simulink subsystem "ElectricalThermalSystem"  (R2025a)
settings: Solver=VariableStepAuto  StartTime=0.0  StopTime=10.0  RelTol=1e-3
undefined symbols (not defined in the file): EnvAirTemp, PlantThrEstCmpPwr, PlntThrAirBpt, PlntThrAirCond, PlntThrAirCp, PlntThrAirCpBpt, PlntThrAirPrand, PlntThrAirRho, PlntThrAirVisc, PlntThrBattDCFlwRatio, PlntThrBattJacLen, PlntThrChArea, PlntThrChDia, PlntThrCoolCond, PlntThrCoolCp, PlntThrCoolCpBpt, PlntThrCoolPrand, PlntThrCoolRho, PlntThrCoolVisc, PlntThrDCJacLen, PlntThrEMJacLen, PlntThrEstCOPLut, PlntThrEstDTLut, PlntThrHeaterMaxPwr, PlntThrPmpDisp, PlntThrPmpHeadP, PlntThrPmpMaxSpd, PlntThrPmpMechEff, PlntThrPmpVolEff, PlntThrRadAirArea, PlntThrRadAirDh, PlntThrRadFanAreaFlw, PlntThrRadFlwCoef, PlntThrRadGapHeight, PlntThrRadLength, PlntThrRadNTubes, PlntThrRadTubeDh, PlntThrRadTubeHeight, PlntThrRadWidth
libraries: autolibutils x62
(part 3 of 4)

== system ElectricalThermalSystem/Heater Battery DCDC Converter/DC-DC Converter/Heat-flow Rate ==
  HTC : Inport
  PwrETemp : Inport  Port=2
  JacArea : Inport  Port=3
  CoolBlkTemp : Inport  Port=4
  Product1 : Product  Inputs=3
  Subtract : Sum  Inputs=+-
  Qpwre : Outport
  wires:
  HTC/1 -> Product1/1
  Product1/1 -> Qpwre/1
  CoolBlkTemp/1 -> Subtract/2
  PwrETemp/1 -> Subtract/1
  Subtract/1 -> Product1/3
  JacArea/1 -> Product1/2

== system ElectricalThermalSystem/Motor/FourEMs/EM1 ==
  CoolTempIn : Inport
  CoolMFlow : Inport  Port=2
  EMTemp : Inport  Port=3
  Constant : Constant  Value=JacHtArea  SampleTime=-1
  Constant1 : Constant  Value=JacDia
  Constant2 : Constant  Value=JacArea
  Constant3 : Constant  Value=JacLen
  HTC Estimator EM : Subsystem
      mask DialogControl Control1 Prompt: Convective Heat Transfer Coefficient (HTC) Estimator
      mask DialogControl Container2 Prompt: Description
      mask DialogControl Control2 Prompt: Assumes turbulent flow through a tube.
      mask DialogControl Control3 Prompt: The Nusselt number (NuD) is calculated with empirical formulas depending on 1/DoL.
      mask DialogControl Control4 Prompt: Where:
      mask DialogControl Control5 Prompt: DoL = hydraulic diameter / tube length
      mask DialogControl Control6 Prompt: When 1/DoL >= 400: NuD = 0.023*ReD^0.8*Pr^0.33
      mask DialogControl Control7 Prompt: Where:
      mask DialogControl Control8 Prompt: Pr: Prandtl number, out of 1D LUT depending on fluid temperature
      mask DialogControl Control9 Prompt: ReD: Reynolds number, calculated. ReD = mdot*hdia/(Ac*aVsc)
      mask DialogControl Control10 Prompt: Where:
      mask DialogControl Control11 Prompt: mdot: mass flow
      mask DialogControl Control12 Prompt: hdia: hydraulic diameter
      mask DialogControl Control13 Prompt: Ac: cross section area
      mask DialogControl Control14 Prompt: aVsc: absolute viscosity, out of 1D LUT depending on fluid temperature
      mask DialogControl Control15 Prompt: When 1/DoL < 400: NuD = 0.36*ReD^0.8*Pr^0.33*DoL^0.055
      mask DialogControl Control16 Prompt: Finally, HTC = k*NuD/hdia
      mask DialogControl Control17 Prompt: Where:
      mask DialogControl Control18 Prompt: k: thermal conductivity, out of 1D LUT depending on fluid temperature
  Temperature and Heat Flow : Subsystem
      mask DialogControl DescTextVar Prompt: Temperature and Heat Flow
      mask DialogControl ParameterGroupVar Prompt: Description
      mask DialogControl Control2 Prompt: Calculates the change in coolant temperature and the heat flow through the EM cooling jacket.
      mask DialogControl Control11 Prompt: Q = HTC*JacA*(Tem-(Tin+Tout)/2)
      mask DialogControl Control3 Prompt: Q = mdot*Cp*(Tout-Tin)
      mask DialogControl Control4 Prompt: Where:
      mask DialogControl Control5 Prompt: Q: heat flow
      mask DialogControl Control12 Prompt: HTC: convective heat transfer coefficient
      mask DialogControl Control13 Prompt: JacA: cooling jacket area
      mask DialogControl Control14 Prompt: Tem: EM temperature
      mask DialogControl Control7 Prompt: mdot: mass flow
      mask DialogControl Control8 Prompt: Cp: heat capacity
      mask DialogControl Control10 Prompt: Tout: coolant temperature (outlet)
      mask DialogControl Control9 Prompt: Tin: coolant temperature (inlet)
  Qem : Outport
  CoolTempOut : Outport  Port=2
  wires:
  Constant/1 -> Temperature and Heat Flow/5(JacArea)
  CoolTempIn/1 -> Temperature and Heat Flow/2(CoolTempIn)
  Temperature and Heat Flow/3(CoolTempOut) -> CoolTempOut/1
  Temperature and Heat Flow/2(Qem) -> Qem/1
  Constant2/1 -> HTC Estimator EM/3(CrossA)
  [BulkCoolTemp] -> HTC Estimator EM/1(FluidTemp)
  Constant3/1 -> HTC Estimator EM/5(TubLen)
  EMTemp/1 -> Temperature and Heat Flow/3(EMTemp)
  [CoolMFlw] -> Temperature and Heat Flow/4(CoolMflw)
  CoolMFlow/1 -> [CoolMFlw], HTC Estimator EM/2(MassFlow)
  HTC Estimator EM/1(HTC) -> Temperature and Heat Flow/1(HTC)
  Temperature and Heat Flow/1(BulkCoolTemp) -> [BulkCoolTemp]
  Constant1/1 -> HTC Estimator EM/4(HydDia)

== system ElectricalThermalSystem/Motor/FourEMs/EM2 ==
  CoolTempIn : Inport
  CoolMFlow : Inport  Port=2
  EMTemp : Inport  Port=3
  Constant : Constant  Value=JacHtArea  SampleTime=-1
  Constant1 : Constant  Value=JacDia
  Constant2 : Constant  Value=JacArea
  Constant3 : Constant  Value=JacLen
  HTC Estimator EM : Subsystem
      mask DialogControl Control1 Prompt: Convective Heat Transfer Coefficient (HTC) Estimator
      mask DialogControl Container2 Prompt: Description
      mask DialogControl Control2 Prompt: Assumes turbulent flow through a tube.
      mask DialogControl Control3 Prompt: The Nusselt number (NuD) is calculated with empirical formulas depending on 1/DoL.
      mask DialogControl Control4 Prompt: Where:
      mask DialogControl Control5 Prompt: DoL = hydraulic diameter / tube length
      mask DialogControl Control6 Prompt: When 1/DoL >= 400: NuD = 0.023*ReD^0.8*Pr^0.33
      mask DialogControl Control7 Prompt: Where:
      mask DialogControl Control8 Prompt: Pr: Prandtl number, out of 1D LUT depending on fluid temperature
      mask DialogControl Control9 Prompt: ReD: Reynolds number, calculated. ReD = mdot*hdia/(Ac*aVsc)
      mask DialogControl Control10 Prompt: Where:
      mask DialogControl Control11 Prompt: mdot: mass flow
      mask DialogControl Control12 Prompt: hdia: hydraulic diameter
      mask DialogControl Control13 Prompt: Ac: cross section area
      mask DialogControl Control14 Prompt: aVsc: absolute viscosity, out of 1D LUT depending on fluid temperature
      mask DialogControl Control15 Prompt: When 1/DoL < 400: NuD = 0.36*ReD^0.8*Pr^0.33*DoL^0.055
      mask DialogControl Control16 Prompt: Finally, HTC = k*NuD/hdia
      mask DialogControl Control17 Prompt: Where:
      mask DialogControl Control18 Prompt: k: thermal conductivity, out of 1D LUT depending on fluid temperature
  Temperature and Heat Flow : Subsystem
      mask DialogControl DescTextVar Prompt: Temperature and Heat Flow
      mask DialogControl ParameterGroupVar Prompt: Description
      mask DialogControl Control2 Prompt: Calculates the change in coolant temperature and the heat flow through the EM cooling jacket.
      mask DialogControl Control11 Prompt: Q = HTC*JacA*(Tem-(Tin+Tout)/2)
      mask DialogControl Control3 Prompt: Q = mdot*Cp*(Tout-Tin)
      mask DialogControl Control4 Prompt: Where:
      mask DialogControl Control5 Prompt: Q: heat flow
      mask DialogControl Control12 Prompt: HTC: convective heat transfer coefficient
      mask DialogControl Control13 Prompt: JacA: cooling jacket area
      mask DialogControl Control14 Prompt: Tem: EM temperature
      mask DialogControl Control7 Prompt: mdot: mass flow
      mask DialogControl Control8 Prompt: Cp: heat capacity
      mask DialogControl Control10 Prompt: Tout: coolant temperature (outlet)
      mask DialogControl Control9 Prompt: Tin: coolant temperature (inlet)
  Qem : Outport
  CoolTempOut : Outport  Port=2
  wires:
  Constant/1 -> Temperature and Heat Flow/5(JacArea)
  CoolTempIn/1 -> Temperature and Heat Flow/2(CoolTempIn)
  Temperature and Heat Flow/3(CoolTempOut) -> CoolTempOut/1
  Temperature and Heat Flow/2(Qem) -> Qem/1
  Constant2/1 -> HTC Estimator EM/3(CrossA)
  [BulkCoolTemp] -> HTC Estimator EM/1(FluidTemp)
  Constant3/1 -> HTC Estimator EM/5(TubLen)
  EMTemp/1 -> Temperature and Heat Flow/3(EMTemp)
  [CoolMFlw] -> Temperature and Heat Flow/4(CoolMflw)
  CoolMFlow/1 -> [CoolMFlw], HTC Estimator EM/2(MassFlow)
  HTC Estimator EM/1(HTC) -> Temperature and Heat Flow/1(HTC)
  Temperature and Heat Flow/1(BulkCoolTemp) -> [BulkCoolTemp]
  Constant1/1 -> HTC Estimator EM/4(HydDia)

== system ElectricalThermalSystem/Motor/FourEMs/EM3 ==
  CoolTempIn : Inport
  CoolMFlow : Inport  Port=2
  EMTemp : Inport  Port=3
  Constant : Constant  Value=JacHtArea  SampleTime=-1
  Constant1 : Constant  Value=JacDia
  Constant2 : Constant  Value=JacArea
  Constant3 : Constant  Value=JacLen
  HTC Estimator EM : Subsystem
      mask DialogControl Control1 Prompt: Convective Heat Transfer Coefficient (HTC) Estimator
      mask DialogControl Container2 Prompt: Description
      mask DialogControl Control2 Prompt: Assumes turbulent flow through a tube.
      mask DialogControl Control3 Prompt: The Nusselt number (NuD) is calculated with empirical formulas depending on 1/DoL.
      mask DialogControl Control4 Prompt: Where:
      mask DialogControl Control5 Prompt: DoL = hydraulic diameter / tube length
      mask DialogControl Control6 Prompt: When 1/DoL >= 400: NuD = 0.023*ReD^0.8*Pr^0.33
      mask DialogControl Control7 Prompt: Where:
      mask DialogControl Control8 Prompt: Pr: Prandtl number, out of 1D LUT depending on fluid temperature
      mask DialogControl Control9 Prompt: ReD: Reynolds number, calculated. ReD = mdot*hdia/(Ac*aVsc)
      mask DialogControl Control10 Prompt: Where:
      mask DialogControl Control11 Prompt: mdot: mass flow
      mask DialogControl Control12 Prompt: hdia: hydraulic diameter
      mask DialogControl Control13 Prompt: Ac: cross section area
      mask DialogControl Control14 Prompt: aVsc: absolute viscosity, out of 1D LUT depending on fluid temperature
      mask DialogControl Control15 Prompt: When 1/DoL < 400: NuD = 0.36*ReD^0.8*Pr^0.33*DoL^0.055
      mask DialogControl Control16 Prompt: Finally, HTC = k*NuD/hdia
      mask DialogControl Control17 Prompt: Where:
      mask DialogControl Control18 Prompt: k: thermal conductivity, out of 1D LUT depending on fluid temperature
  Temperature and Heat Flow : Subsystem
      mask DialogControl DescTextVar Prompt: Temperature and Heat Flow
      mask DialogControl ParameterGroupVar Prompt: Description
      mask DialogControl Control2 Prompt: Calculates the change in coolant temperature and the heat flow through the EM cooling jacket.
      mask DialogControl Control11 Prompt: Q = HTC*JacA*(Tem-(Tin+Tout)/2)
      mask DialogControl Control3 Prompt: Q = mdot*Cp*(Tout-Tin)
      mask DialogControl Control4 Prompt: Where:
      mask DialogControl Control5 Prompt: Q: heat flow
      mask DialogControl Control12 Prompt: HTC: convective heat transfer coefficient
      mask DialogControl Control13 Prompt: JacA: cooling jacket area
      mask DialogControl Control14 Prompt: Tem: EM temperature
      mask DialogControl Control7 Prompt: mdot: mass flow
      mask DialogControl Control8 Prompt: Cp: heat capacity
      mask DialogControl Control10 Prompt: Tout: coolant temperature (outlet)
      mask DialogControl Control9 Prompt: Tin: coolant temperature (inlet)
  Qem : Outport
  CoolTempOut : Outport  Port=2
  wires:
  Constant/1 -> Temperature and Heat Flow/5(JacArea)
  CoolTempIn/1 -> Temperature and Heat Flow/2(CoolTempIn)
  Temperature and Heat Flow/3(CoolTempOut) -> CoolTempOut/1
  Temperature and Heat Flow/2(Qem) -> Qem/1
  Constant2/1 -> HTC Estimator EM/3(CrossA)
  [BulkCoolTemp] -> HTC Estimator EM/1(FluidTemp)
  Constant3/1 -> HTC Estimator EM/5(TubLen)
  EMTemp/1 -> Temperature and Heat Flow/3(EMTemp)
  [CoolMFlw] -> Temperature and Heat Flow/4(CoolMflw)
  CoolMFlow/1 -> [CoolMFlw], HTC Estimator EM/2(MassFlow)
  HTC Estimator EM/1(HTC) -> Temperature and Heat Flow/1(HTC)
  Temperature and Heat Flow/1(BulkCoolTemp) -> [BulkCoolTemp]
  Constant1/1 -> HTC Estimator EM/4(HydDia)

== system ElectricalThermalSystem/Motor/FourEMs/EM4 ==
  CoolTempIn : Inport
  CoolMFlow : Inport  Port=2
  EMTemp : Inport  Port=3
  Constant : Constant  Value=JacHtArea  SampleTime=-1
  Constant1 : Constant  Value=JacDia
  Constant2 : Constant  Value=JacArea
  Constant3 : Constant  Value=JacLen
  HTC Estimator EM : Subsystem
      mask DialogControl Control1 Prompt: Convective Heat Transfer Coefficient (HTC) Estimator
      mask DialogControl Container2 Prompt: Description
      mask DialogControl Control2 Prompt: Assumes turbulent flow through a tube.
      mask DialogControl Control3 Prompt: The Nusselt number (NuD) is calculated with empirical formulas depending on 1/DoL.
      mask DialogControl Control4 Prompt: Where:
      mask DialogControl Control5 Prompt: DoL = hydraulic diameter / tube length
      mask DialogControl Control6 Prompt: When 1/DoL >= 400: NuD = 0.023*ReD^0.8*Pr^0.33
      mask DialogControl Control7 Prompt: Where:
      mask DialogControl Control8 Prompt: Pr: Prandtl number, out of 1D LUT depending on fluid temperature
      mask DialogControl Control9 Prompt: ReD: Reynolds number, calculated. ReD = mdot*hdia/(Ac*aVsc)
      mask DialogControl Control10 Prompt: Where:
      mask DialogControl Control11 Prompt: mdot: mass flow
      mask DialogControl Control12 Prompt: hdia: hydraulic diameter
      mask DialogControl Control13 Prompt: Ac: cross section area
      mask DialogControl Control14 Prompt: aVsc: absolute viscosity, out of 1D LUT depending on fluid temperature
      mask DialogControl Control15 Prompt: When 1/DoL < 400: NuD = 0.36*ReD^0.8*Pr^0.33*DoL^0.055
      mask DialogControl Control16 Prompt: Finally, HTC = k*NuD/hdia
      mask DialogControl Control17 Prompt: Where:
      mask DialogControl Control18 Prompt: k: thermal conductivity, out of 1D LUT depending on fluid temperature
  Temperature and Heat Flow : Subsystem
      mask DialogControl DescTextVar Prompt: Temperature and Heat Flow
      mask DialogControl ParameterGroupVar Prompt: Description
      mask DialogControl Control2 Prompt: Calculates the change in coolant temperature and the heat flow through the EM cooling jacket.
      mask DialogControl Control11 Prompt: Q = HTC*JacA*(Tem-(Tin+Tout)/2)
      mask DialogControl Control3 Prompt: Q = mdot*Cp*(Tout-Tin)
      mask DialogControl Control4 Prompt: Where:
      mask DialogControl Control5 Prompt: Q: heat flow
      mask DialogControl Control12 Prompt: HTC: convective heat transfer coefficient
      mask DialogControl Control13 Prompt: JacA: cooling jacket area
      mask DialogControl Control14 Prompt: Tem: EM temperature
      mask DialogControl Control7 Prompt: mdot: mass flow
      mask DialogControl Control8 Prompt: Cp: heat capacity
      mask DialogControl Control10 Prompt: Tout: coolant temperature (outlet)
      mask DialogControl Control9 Prompt: Tin: coolant temperature (inlet)
  Qem : Outport
  CoolTempOut : Outport  Port=2
  wires:
  Constant/1 -> Temperature and Heat Flow/5(JacArea)
  CoolTempIn/1 -> Temperature and Heat Flow/2(CoolTempIn)
  Temperature and Heat Flow/3(CoolTempOut) -> CoolTempOut/1
  Temperature and Heat Flow/2(Qem) -> Qem/1
  Constant2/1 -> HTC Estimator EM/3(CrossA)
  [BulkCoolTemp] -> HTC Estimator EM/1(FluidTemp)
  Constant3/1 -> HTC Estimator EM/5(TubLen)
  EMTemp/1 -> Temperature and Heat Flow/3(EMTemp)
  [CoolMFlw] -> Temperature and Heat Flow/4(CoolMflw)
  CoolMFlow/1 -> [CoolMFlw], HTC Estimator EM/2(MassFlow)
  HTC Estimator EM/1(HTC) -> Temperature and Heat Flow/1(HTC)
  Temperature and Heat Flow/1(BulkCoolTemp) -> [BulkCoolTemp]
  Constant1/1 -> HTC Estimator EM/4(HydDia)

== system ElectricalThermalSystem/Motor/OneEM/EM1 ==
  MassFlow : Inport
  CoolTempIn : Inport  Port=2
  EMTemp : Inport  Port=3
  Constant : Constant  Value=JacHtArea  SampleTime=-1
  Constant1 : Constant  Value=JacDia
  Constant2 : Constant  Value=JacArea
  Constant3 : Constant  Value=JacLen
  HTC Estimator EM : Subsystem
      mask DialogControl Control1 Prompt: Convective Heat Transfer Coefficient (HTC) Estimator
      mask DialogControl Container2 Prompt: Description
      mask DialogControl Control2 Prompt: Assumes turbulent flow through a tube.
      mask DialogControl Control3 Prompt: The Nusselt number (NuD) is calculated with empirical formulas depending on 1/DoL.
      mask DialogControl Control4 Prompt: Where:
      mask DialogControl Control5 Prompt: DoL = hydraulic diameter / tube length
      mask DialogControl Control6 Prompt: When 1/DoL >= 400: NuD = 0.023*ReD^0.8*Pr^0.33
      mask DialogControl Control7 Prompt: Where:
      mask DialogControl Control8 Prompt: Pr: Prandtl number, out of 1D LUT depending on fluid temperature
      mask DialogControl Control9 Prompt: ReD: Reynolds number, calculated. ReD = mdot*hdia/(Ac*aVsc)
      mask DialogControl Control10 Prompt: Where:
      mask DialogControl Control11 Prompt: mdot: mass flow
      mask DialogControl Control12 Prompt: hdia: hydraulic diameter
      mask DialogControl Control13 Prompt: Ac: cross section area
      mask DialogControl Control14 Prompt: aVsc: absolute viscosity, out of 1D LUT depending on fluid temperature
      mask DialogControl Control15 Prompt: When 1/DoL < 400: NuD = 0.36*ReD^0.8*Pr^0.33*DoL^0.055
      mask DialogControl Control16 Prompt: Finally, HTC = k*NuD/hdia
      mask DialogControl Control17 Prompt: Where:
      mask DialogControl Control18 Prompt: k: thermal conductivity, out of 1D LUT depending on fluid temperature
  Temperature and Heat Flow : Subsystem
      mask DialogControl DescTextVar Prompt: Temperature and Heat Flow
      mask DialogControl ParameterGroupVar Prompt: Description
      mask DialogControl Control2 Prompt: Calculates the change in coolant temperature and the heat flow through the EM cooling jacket.
      mask DialogControl Control11 Prompt: Q = HTC*JacA*(Tem-(Tin+Tout)/2)
      mask DialogControl Control3 Prompt: Q = mdot*Cp*(Tout-Tin)
      mask DialogControl Control4 Prompt: Where:
      mask DialogControl Control5 Prompt: Q: heat flow
      mask DialogControl Control12 Prompt: HTC: convective heat transfer coefficient
      mask DialogControl Control13 Prompt: JacA: cooling jacket area
      mask DialogControl Control14 Prompt: Tem: EM temperature
      mask DialogControl Control7 Prompt: mdot: mass flow
      mask DialogControl Control8 Prompt: Cp: heat capacity
      mask DialogControl Control10 Prompt: Tout: coolant temperature (outlet)
      mask DialogControl Control9 Prompt: Tin: coolant temperature (inlet)
  Qem : Outport
  CoolTempOut : Outport  Port=2
  wires:
  Constant/1 -> Temperature and Heat Flow/5(JacArea)
  CoolTempIn/1 -> Temperature and Heat Flow/2(CoolTempIn)
  Temperature and Heat Flow/3(CoolTempOut) -> CoolTempOut/1
  Temperature and Heat Flow/2(Qem) -> Qem/1
  Constant2/1 -> HTC Estimator EM/3(CrossA)
  [BulkCoolTemp] -> HTC Estimator EM/1(FluidTemp)
  Constant3/1 -> HTC Estimator EM/5(TubLen)
  EMTemp/1 -> Temperature and Heat Flow/3(EMTemp)
  [CoolMFlw] -> Temperature and Heat Flow/4(CoolMflw)
  MassFlow/1 -> [CoolMFlw], HTC Estimator EM/2(MassFlow)
  HTC Estimator EM/1(HTC) -> Temperature and Heat Flow/1(HTC)
  Temperature and Heat Flow/1(BulkCoolTemp) -> [BulkCoolTemp]
  Constant1/1 -> HTC Estimator EM/4(HydDia)

== system ElectricalThermalSystem/Motor/ThreeEMs/EM1 ==
  CoolTempIn : Inport
  CoolMFlow : Inport  Port=2
  EMTemp : Inport  Port=3
  Constant : Constant  Value=JacHtArea  SampleTime=-1
  Constant1 : Constant  Value=JacDia
  Constant2 : Constant  Value=JacArea
  Constant3 : Constant  Value=JacLen
  HTC Estimator EM : Subsystem
      mask DialogControl Control1 Prompt: Convective Heat Transfer Coefficient (HTC) Estimator
      mask DialogControl Container2 Prompt: Description
      mask DialogControl Control2 Prompt: Assumes turbulent flow through a tube.
      mask DialogControl Control3 Prompt: The Nusselt number (NuD) is calculated with empirical formulas depending on 1/DoL.
      mask DialogControl Control4 Prompt: Where:
      mask DialogControl Control5 Prompt: DoL = hydraulic diameter / tube length
      mask DialogControl Control6 Prompt: When 1/DoL >= 400: NuD = 0.023*ReD^0.8*Pr^0.33
      mask DialogControl Control7 Prompt: Where:
      mask DialogControl Control8 Prompt: Pr: Prandtl number, out of 1D LUT depending on fluid temperature
      mask DialogControl Control9 Prompt: ReD: Reynolds number, calculated. ReD = mdot*hdia/(Ac*aVsc)
      mask DialogControl Control10 Prompt: Where:
      mask DialogControl Control11 Prompt: mdot: mass flow
      mask DialogControl Control12 Prompt: hdia: hydraulic diameter
      mask DialogControl Control13 Prompt: Ac: cross section area
      mask DialogControl Control14 Prompt: aVsc: absolute viscosity, out of 1D LUT depending on fluid temperature
      mask DialogControl Control15 Prompt: When 1/DoL < 400: NuD = 0.36*ReD^0.8*Pr^0.33*DoL^0.055
      mask DialogControl Control16 Prompt: Finally, HTC = k*NuD/hdia
      mask DialogControl Control17 Prompt: Where:
      mask DialogControl Control18 Prompt: k: thermal conductivity, out of 1D LUT depending on fluid temperature
  Temperature and Heat Flow : Subsystem
      mask DialogControl DescTextVar Prompt: Temperature and Heat Flow
      mask DialogControl ParameterGroupVar Prompt: Description
      mask DialogControl Control2 Prompt: Calculates the change in coolant temperature and the heat flow through the EM cooling jacket.
      mask DialogControl Control11 Prompt: Q = HTC*JacA*(Tem-(Tin+Tout)/2)
      mask DialogControl Control3 Prompt: Q = mdot*Cp*(Tout-Tin)
      mask DialogControl Control4 Prompt: Where:
      mask DialogControl Control5 Prompt: Q: heat flow
      mask DialogControl Control12 Prompt: HTC: convective heat transfer coefficient
      mask DialogControl Control13 Prompt: JacA: cooling jacket area
      mask DialogControl Control14 Prompt: Tem: EM temperature
      mask DialogControl Control7 Prompt: mdot: mass flow
      mask DialogControl Control8 Prompt: Cp: heat capacity
      mask DialogControl Control10 Prompt: Tout: coolant temperature (outlet)
      mask DialogControl Control9 Prompt: Tin: coolant temperature (inlet)
  Qem : Outport
  CoolTempOut : Outport  Port=2
  wires:
  Constant/1 -> Temperature and Heat Flow/5(JacArea)
  CoolTempIn/1 -> Temperature and Heat Flow/2(CoolTempIn)
  Temperature and Heat Flow/3(CoolTempOut) -> CoolTempOut/1
  Temperature and Heat Flow/2(Qem) -> Qem/1
  Constant2/1 -> HTC Estimator EM/3(CrossA)
  [BulkCoolTemp] -> HTC Estimator EM/1(FluidTemp)
  Constant3/1 -> HTC Estimator EM/5(TubLen)
  EMTemp/1 -> Temperature and Heat Flow/3(EMTemp)
  [CoolMFlw] -> Temperature and Heat Flow/4(CoolMflw)
  CoolMFlow/1 -> [CoolMFlw], HTC Estimator EM/2(MassFlow)
  HTC Estimator EM/1(HTC) -> Temperature and Heat Flow/1(HTC)
  Temperature and Heat Flow/1(BulkCoolTemp) -> [BulkCoolTemp]
  Constant1/1 -> HTC Estimator EM/4(HydDia)

== system ElectricalThermalSystem/Motor/ThreeEMs/EM2 ==
  CoolTempIn : Inport
  CoolMFlow : Inport  Port=2
  EMTemp : Inport  Port=3
  Constant : Constant  Value=JacHtArea  SampleTime=-1
  Constant1 : Constant  Value=JacDia
  Constant2 : Constant  Value=JacArea
  Constant3 : Constant  Value=JacLen
  HTC Estimator EM : Subsystem
      mask DialogControl Control1 Prompt: Convective Heat Transfer Coefficient (HTC) Estimator
      mask DialogControl Container2 Prompt: Description
      mask DialogControl Control2 Prompt: Assumes turbulent flow through a tube.
      mask DialogControl Control3 Prompt: The Nusselt number (NuD) is calculated with empirical formulas depending on 1/DoL.
      mask DialogControl Control4 Prompt: Where:
      mask DialogControl Control5 Prompt: DoL = hydraulic diameter / tube length
      mask DialogControl Control6 Prompt: When 1/DoL >= 400: NuD = 0.023*ReD^0.8*Pr^0.33
      mask DialogControl Control7 Prompt: Where:
      mask DialogControl Control8 Prompt: Pr: Prandtl number, out of 1D LUT depending on fluid temperature
      mask DialogControl Control9 Prompt: ReD: Reynolds number, calculated. ReD = mdot*hdia/(Ac*aVsc)
      mask DialogControl Control10 Prompt: Where:
      mask DialogControl Control11 Prompt: mdot: mass flow
      mask DialogControl Control12 Prompt: hdia: hydraulic diameter
      mask DialogControl Control13 Prompt: Ac: cross section area
      mask DialogControl Control14 Prompt: aVsc: absolute viscosity, out of 1D LUT depending on fluid temperature
      mask DialogControl Control15 Prompt: When 1/DoL < 400: NuD = 0.36*ReD^0.8*Pr^0.33*DoL^0.055
      mask DialogControl Control16 Prompt: Finally, HTC = k*NuD/hdia
      mask DialogControl Control17 Prompt: Where:
      mask DialogControl Control18 Prompt: k: thermal conductivity, out of 1D LUT depending on fluid temperature
  Temperature and Heat Flow : Subsystem
      mask DialogControl DescTextVar Prompt: Temperature and Heat Flow
      mask DialogControl ParameterGroupVar Prompt: Description
      mask DialogControl Control2 Prompt: Calculates the change in coolant temperature and the heat flow through the EM cooling jacket.
      mask DialogControl Control11 Prompt: Q = HTC*JacA*(Tem-(Tin+Tout)/2)
      mask DialogControl Control3 Prompt: Q = mdot*Cp*(Tout-Tin)
      mask DialogControl Control4 Prompt: Where:
      mask DialogControl Control5 Prompt: Q: heat flow
      mask DialogControl Control12 Prompt: HTC: convective heat transfer coefficient
      mask DialogControl Control13 Prompt: JacA: cooling jacket area
      mask DialogControl Control14 Prompt: Tem: EM temperature
      mask DialogControl Control7 Prompt: mdot: mass flow
      mask DialogControl Control8 Prompt: Cp: heat capacity
      mask DialogControl Control10 Prompt: Tout: coolant temperature (outlet)
      mask DialogControl Control9 Prompt: Tin: coolant temperature (inlet)
  Qem : Outport
  CoolTempOut : Outport  Port=2
  wires:
  Constant/1 -> Temperature and Heat Flow/5(JacArea)
  CoolTempIn/1 -> Temperature and Heat Flow/2(CoolTempIn)
  Temperature and Heat Flow/3(CoolTempOut) -> CoolTempOut/1
  Temperature and Heat Flow/2(Qem) -> Qem/1
  Constant2/1 -> HTC Estimator EM/3(CrossA)
  [BulkCoolTemp] -> HTC Estimator EM/1(FluidTemp)
  Constant3/1 -> HTC Estimator EM/5(TubLen)
  EMTemp/1 -> Temperature and Heat Flow/3(EMTemp)
  [CoolMFlw] -> Temperature and Heat Flow/4(CoolMflw)
  CoolMFlow/1 -> [CoolMFlw], HTC Estimator EM/2(MassFlow)
  HTC Estimator EM/1(HTC) -> Temperature and Heat Flow/1(HTC)
  Temperature and Heat Flow/1(BulkCoolTemp) -> [BulkCoolTemp]
  Constant1/1 -> HTC Estimator EM/4(HydDia)

== system ElectricalThermalSystem/Motor/ThreeEMs/EM3 ==
  CoolTempIn : Inport
  CoolMFlow : Inport  Port=2
  EMTemp : Inport  Port=3
  Constant : Constant  Value=JacHtArea  SampleTime=-1
  Constant1 : Constant  Value=JacDia
  Constant2 : Constant  Value=JacArea
  Constant3 : Constant  Value=JacLen
  HTC Estimator EM : Subsystem
      mask DialogControl Control1 Prompt: Convective Heat Transfer Coefficient (HTC) Estimator
      mask DialogControl Container2 Prompt: Description
      mask DialogControl Control2 Prompt: Assumes turbulent flow through a tube.
      mask DialogControl Control3 Prompt: The Nusselt number (NuD) is calculated with empirical formulas depending on 1/DoL.
      mask DialogControl Control4 Prompt: Where:
      mask DialogControl Control5 Prompt: DoL = hydraulic diameter / tube length
      mask DialogControl Control6 Prompt: When 1/DoL >= 400: NuD = 0.023*ReD^0.8*Pr^0.33
      mask DialogControl Control7 Prompt: Where:
      mask DialogControl Control8 Prompt: Pr: Prandtl number, out of 1D LUT depending on fluid temperature
      mask DialogControl Control9 Prompt: ReD: Reynolds number, calculated. ReD = mdot*hdia/(Ac*aVsc)
      mask DialogControl Control10 Prompt: Where:
      mask DialogControl Control11 Prompt: mdot: mass flow
      mask DialogControl Control12 Prompt: hdia: hydraulic diameter
      mask DialogControl Control13 Prompt: Ac: cross section area
      mask DialogControl Control14 Prompt: aVsc: absolute viscosity, out of 1D LUT depending on fluid temperature
      mask DialogControl Control15 Prompt: When 1/DoL < 400: NuD = 0.36*ReD^0.8*Pr^0.33*DoL^0.055
      mask DialogControl Control16 Prompt: Finally, HTC = k*NuD/hdia
      mask DialogControl Control17 Prompt: Where:
      mask DialogControl Control18 Prompt: k: thermal conductivity, out of 1D LUT depending on fluid temperature
  Temperature and Heat Flow : Subsystem
      mask DialogControl DescTextVar Prompt: Temperature and Heat Flow
      mask DialogControl ParameterGroupVar Prompt: Description
      mask DialogControl Control2 Prompt: Calculates the change in coolant temperature and the heat flow through the EM cooling jacket.
      mask DialogControl Control11 Prompt: Q = HTC*JacA*(Tem-(Tin+Tout)/2)
      mask DialogControl Control3 Prompt: Q = mdot*Cp*(Tout-Tin)
      mask DialogControl Control4 Prompt: Where:
      mask DialogControl Control5 Prompt: Q: heat flow
      mask DialogControl Control12 Prompt: HTC: convective heat transfer coefficient
      mask DialogControl Control13 Prompt: JacA: cooling jacket area
      mask DialogControl Control14 Prompt: Tem: EM temperature
      mask DialogControl Control7 Prompt: mdot: mass flow
      mask DialogControl Control8 Prompt: Cp: heat capacity
      mask DialogControl Control10 Prompt: Tout: coolant temperature (outlet)
      mask DialogControl Control9 Prompt: Tin: coolant temperature (inlet)
  Qem : Outport
  CoolTempOut : Outport  Port=2
  wires:
  Constant/1 -> Temperature and Heat Flow/5(JacArea)
  CoolTempIn/1 -> Temperature and Heat Flow/2(CoolTempIn)
  Temperature and Heat Flow/3(CoolTempOut) -> CoolTempOut/1
  Temperature and Heat Flow/2(Qem) -> Qem/1
  Constant2/1 -> HTC Estimator EM/3(CrossA)
  [BulkCoolTemp] -> HTC Estimator EM/1(FluidTemp)
  Constant3/1 -> HTC Estimator EM/5(TubLen)
  EMTemp/1 -> Temperature and Heat Flow/3(EMTemp)
  [CoolMFlw] -> Temperature and Heat Flow/4(CoolMflw)
  CoolMFlow/1 -> [CoolMFlw], HTC Estimator EM/2(MassFlow)
  HTC Estimator EM/1(HTC) -> Temperature and Heat Flow/1(HTC)
  Temperature and Heat Flow/1(BulkCoolTemp) -> [BulkCoolTemp]
  Constant1/1 -> HTC Estimator EM/4(HydDia)

== system ElectricalThermalSystem/Motor/TwoEMs/EM1 ==
  CoolTempIn : Inport
  CoolMFlow : Inport  Port=2
  EMTemp : Inport  Port=3
  Constant : Constant  Value=JacHtArea  SampleTime=-1
  Constant1 : Constant  Value=JacDia
  Constant2 : Constant  Value=JacArea
  Constant3 : Constant  Value=JacLen
  HTC Estimator EM : Subsystem
      mask DialogControl Control1 Prompt: Convective Heat Transfer Coefficient (HTC) Estimator
      mask DialogControl Container2 Prompt: Description
      mask DialogControl Control2 Prompt: Assumes turbulent flow through a tube.
      mask DialogControl Control3 Prompt: The Nusselt number (NuD) is calculated with empirical formulas depending on 1/DoL.
      mask DialogControl Control4 Prompt: Where:
      mask DialogControl Control5 Prompt: DoL = hydraulic diameter / tube length
      mask DialogControl Control6 Prompt: When 1/DoL >= 400: NuD = 0.023*ReD^0.8*Pr^0.33
      mask DialogControl Control7 Prompt: Where:
      mask DialogControl Control8 Prompt: Pr: Prandtl number, out of 1D LUT depending on fluid temperature
      mask DialogControl Control9 Prompt: ReD: Reynolds number, calculated. ReD = mdot*hdia/(Ac*aVsc)
      mask DialogControl Control10 Prompt: Where:
      mask DialogControl Control11 Prompt: mdot: mass flow
      mask DialogControl Control12 Prompt: hdia: hydraulic diameter
      mask DialogControl Control13 Prompt: Ac: cross section area
      mask DialogControl Control14 Prompt: aVsc: absolute viscosity, out of 1D LUT depending on fluid temperature
      mask DialogControl Control15 Prompt: When 1/DoL < 400: NuD = 0.36*ReD^0.8*Pr^0.33*DoL^0.055
      mask DialogControl Control16 Prompt: Finally, HTC = k*NuD/hdia
      mask DialogControl Control17 Prompt: Where:
      mask DialogControl Control18 Prompt: k: thermal conductivity, out of 1D LUT depending on fluid temperature
  Temperature and Heat Flow : Subsystem
      mask DialogControl DescTextVar Prompt: Temperature and Heat Flow
      mask DialogControl ParameterGroupVar Prompt: Description
      mask DialogControl Control2 Prompt: Calculates the change in coolant temperature and the heat flow through the EM cooling jacket.
      mask DialogControl Control11 Prompt: Q = HTC*JacA*(Tem-(Tin+Tout)/2)
      mask DialogControl Control3 Prompt: Q = mdot*Cp*(Tout-Tin)
      mask DialogControl Control4 Prompt: Where:
      mask DialogControl Control5 Prompt: Q: heat flow
      mask DialogControl Control12 Prompt: HTC: convective heat transfer coefficient
      mask DialogControl Control13 Prompt: JacA: cooling jacket area
      mask DialogControl Control14 Prompt: Tem: EM temperature
      mask DialogControl Control7 Prompt: mdot: mass flow
      mask DialogControl Control8 Prompt: Cp: heat capacity
      mask DialogControl Control10 Prompt: Tout: coolant temperature (outlet)
      mask DialogControl Control9 Prompt: Tin: coolant temperature (inlet)
  Qem : Outport
  CoolTempOut : Outport  Port=2
  wires:
  Constant/1 -> Temperature and Heat Flow/5(JacArea)
  CoolTempIn/1 -> Temperature and Heat Flow/2(CoolTempIn)
  Temperature and Heat Flow/3(CoolTempOut) -> CoolTempOut/1
  Temperature and Heat Flow/2(Qem) -> Qem/1
  Constant2/1 -> HTC Estimator EM/3(CrossA)
  [BulkCoolTemp] -> HTC Estimator EM/1(FluidTemp)
  Constant3/1 -> HTC Estimator EM/5(TubLen)
  EMTemp/1 -> Temperature and Heat Flow/3(EMTemp)
  [CoolMFlw] -> Temperature and Heat Flow/4(CoolMflw)
  CoolMFlow/1 -> [CoolMFlw], HTC Estimator EM/2(MassFlow)
  HTC Estimator EM/1(HTC) -> Temperature and Heat Flow/1(HTC)
  Temperature and Heat Flow/1(BulkCoolTemp) -> [BulkCoolTemp]
  Constant1/1 -> HTC Estimator EM/4(HydDia)

== system ElectricalThermalSystem/Motor/TwoEMs/EM2 ==
  CoolTempIn : Inport
  CoolMFlow : Inport  Port=2
  EMTemp : Inport  Port=3
  Constant : Constant  Value=JacHtArea  SampleTime=-1
  Constant1 : Constant  Value=JacDia
  Constant2 : Constant  Value=JacArea
  Constant3 : Constant  Value=JacLen
  HTC Estimator EM : Subsystem
      mask DialogControl Control1 Prompt: Convective Heat Transfer Coefficient (HTC) Estimator
      mask DialogControl Container2 Prompt: Description
      mask DialogControl Control2 Prompt: Assumes turbulent flow through a tube.
      mask DialogControl Control3 Prompt: The Nusselt number (NuD) is calculated with empirical formulas depending on 1/DoL.
      mask DialogControl Control4 Prompt: Where:
      mask DialogControl Control5 Prompt: DoL = hydraulic diameter / tube length
      mask DialogControl Control6 Prompt: When 1/DoL >= 400: NuD = 0.023*ReD^0.8*Pr^0.33
      mask DialogControl Control7 Prompt: Where:
      mask DialogControl Control8 Prompt: Pr: Prandtl number, out of 1D LUT depending on fluid temperature
      mask DialogControl Control9 Prompt: ReD: Reynolds number, calculated. ReD = mdot*hdia/(Ac*aVsc)
      mask DialogControl Control10 Prompt: Where:
      mask DialogControl Control11 Prompt: mdot: mass flow
      mask DialogControl Control12 Prompt: hdia: hydraulic diameter
      mask DialogControl Control13 Prompt: Ac: cross section area
      mask DialogControl Control14 Prompt: aVsc: absolute viscosity, out of 1D LUT depending on fluid temperature
      mask DialogControl Control15 Prompt: When 1/DoL < 400: NuD = 0.36*ReD^0.8*Pr^0.33*DoL^0.055
      mask DialogControl Control16 Prompt: Finally, HTC = k*NuD/hdia
      mask DialogControl Control17 Prompt: Where:
      mask DialogControl Control18 Prompt: k: thermal conductivity, out of 1D LUT depending on fluid temperature
  Temperature and Heat Flow : Subsystem
      mask DialogControl DescTextVar Prompt: Temperature and Heat Flow
      mask DialogControl ParameterGroupVar Prompt: Description
      mask DialogControl Control2 Prompt: Calculates the change in coolant temperature and the heat flow through the EM cooling jacket.
      mask DialogControl Control11 Prompt: Q = HTC*JacA*(Tem-(Tin+Tout)/2)
      mask DialogControl Control3 Prompt: Q = mdot*Cp*(Tout-Tin)
      mask DialogControl Control4 Prompt: Where:
      mask DialogControl Control5 Prompt: Q: heat flow
      mask DialogControl Control12 Prompt: HTC: convective heat transfer coefficient
      mask DialogControl Control13 Prompt: JacA: cooling jacket area
      mask DialogControl Control14 Prompt: Tem: EM temperature
      mask DialogControl Control7 Prompt: mdot: mass flow
      mask DialogControl Control8 Prompt: Cp: heat capacity
      mask DialogControl Control10 Prompt: Tout: coolant temperature (outlet)
      mask DialogControl Control9 Prompt: Tin: coolant temperature (inlet)
  Qem : Outport
  CoolTempOut : Outport  Port=2
  wires:
  Constant/1 -> Temperature and Heat Flow/5(JacArea)
  CoolTempIn/1 -> Temperature and Heat Flow/2(CoolTempIn)
  Temperature and Heat Flow/3(CoolTempOut) -> CoolTempOut/1
  Temperature and Heat Flow/2(Qem) -> Qem/1
  Constant2/1 -> HTC Estimator EM/3(CrossA)
  [BulkCoolTemp] -> HTC Estimator EM/1(FluidTemp)
  Constant3/1 -> HTC Estimator EM/5(TubLen)
  EMTemp/1 -> Temperature and Heat Flow/3(EMTemp)
  [CoolMFlw] -> Temperature and Heat Flow/4(CoolMflw)
  CoolMFlow/1 -> [CoolMFlw], HTC Estimator EM/2(MassFlow)
  HTC Estimator EM/1(HTC) -> Temperature and Heat Flow/1(HTC)
  Temperature and Heat Flow/1(BulkCoolTemp) -> [BulkCoolTemp]
  Constant1/1 -> HTC Estimator EM/4(HydDia)

== system ElectricalThermalSystem/Refrigeration Loop/Chiller Coolant Temperature/LPF with IC3 ==
  u : Inport
  Cont LPF IC : autolibutils/Cont LPF IC  wc=wc  aMode=1  dataType=off
  Initial Condition : Constant  Value=InitCond  SampleTime=-1
  y : Outport
  wires:
  Cont LPF IC/1 -> y/1
  u/1 -> Cont LPF IC/1
  Initial Condition/1 -> Cont LPF IC/2

== system ElectricalThermalSystem/Refrigeration Loop/Heat-flow Rate and Power/LPF with IC1 ==
  u : Inport
  Cont LPF IC : autolibutils/Cont LPF IC  wc=wc  aMode=1  dataType=off
  Initial Condition : Constant  Value=InitCond  SampleTime=-1
  y : Outport
  wires:
  Cont LPF IC/1 -> y/1
  u/1 -> Cont LPF IC/1
  Initial Condition/1 -> Cont LPF IC/2

== system ElectricalThermalSystem/Front Side HXs/Radiator/Air Temperature/LPF with IC1 ==
  u : Inport
  Cont LPF IC : autolibutils/Cont LPF IC  wc=wc  aMode=1  dataType=off
  Initial Condition : Constant  Value=InitCond  SampleTime=-1
  y : Outport
  wires:
  Cont LPF IC/1 -> y/1
  u/1 -> Cont LPF IC/1
  Initial Condition/1 -> Cont LPF IC/2

== system ElectricalThermalSystem/Front Side HXs/Radiator/Coolant Temperature/LPF Temperature ==
  u : Inport
  Cont LPF IC : autolibutils/Cont LPF IC  wc=wc  aMode=1  dataType=off
  Initial Condition : Constant  Value=InitCond  SampleTime=-1
  y : Outport
  wires:
  Cont LPF IC/1 -> y/1
  u/1 -> Cont LPF IC/1
  Initial Condition/1 -> Cont LPF IC/2

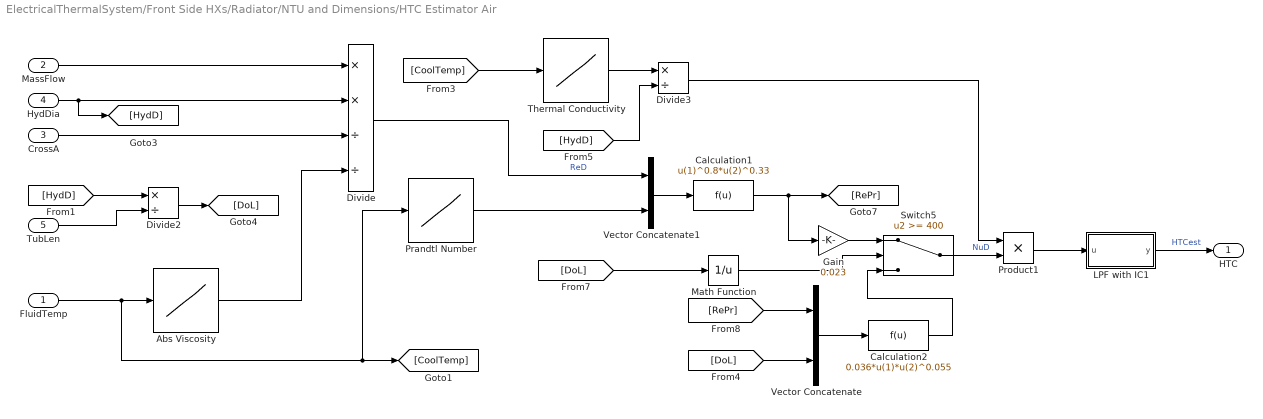
== system ElectricalThermalSystem/Front Side HXs/Radiator/NTU and Dimensions/HTC Estimator Air ==
  FluidTemp : Inport
  MassFlow : Inport  Port=2
  CrossA : Inport  Port=3  OutMin=eps
  HydDia : Inport  Port=4
  TubLen : Inport  Port=5
  Abs Viscosity : Lookup_n-D  NumberOfTableDimensions=1  BreakpointsForDimension1=PlntThrAirCpBpt  Table=PlntThrAirVisc  ExtrapMethod=Clip  UseLastTableValue=on  InternalRulePriority=Speed  RndMeth=Simplest
  Calculation1 : Fcn  Expr=u(1)^0.8*u(2)^0.33
  Calculation2 : Fcn  Expr=0.036*u(1)*u(2)^0.055
  Divide : Product  Inputs=**//
  Divide2 : Product  Inputs=*/
  Divide3 : Product  Inputs=*/
  Gain : Gain  Gain=0.023
  LPF with IC1 : Subsystem  mask{wc=10, InitCond=10, dataType=off}
      mask prompts: wc "Cutoff frequency, wc [rad/s]"; InitCond "Initial condition, InitCond [same as u]"; dataType "Enforce same input data type"
      mask TypeOptions wc: Cont LPF IC/wc
      mask TypeOptions InitCond: Initial Condition/Value
      mask TypeOptions dataType: Cont LPF IC/dataType
  Math Function : Math  Operator=reciprocal
  Prandtl Number : Lookup_n-D  NumberOfTableDimensions=1  BreakpointsForDimension1=PlntThrAirCpBpt  Table=PlntThrAirPrand  ExtrapMethod=Clip  UseLastTableValue=on  InternalRulePriority=Speed  RndMeth=Simplest
  Product1 : Product
  Switch5 : Switch  Threshold=400  SaturateOnIntegerOverflow=off  InputSameDT=off
  Thermal Conductivity : Lookup_n-D  NumberOfTableDimensions=1  BreakpointsForDimension1=PlntThrAirCpBpt  Table=PlntThrAirCond  ExtrapMethod=Clip  UseLastTableValue=on  InternalRulePriority=Speed  RndMeth=Simplest
  Vector Concatenate : Concatenate
  Vector Concatenate1 : Concatenate
  HTC : Outport
  wires:
  MassFlow/1 -> Divide/1
  Product1/1 -> LPF with IC1/1(u)
  Switch5/1 -> Product1/2  "NuD"
  Calculation2/1 -> Switch5/3
  Vector Concatenate/1 -> Calculation2/1
  [DoL] -> Vector Concatenate/2
  [RePr] -> Vector Concatenate/1
  Calculation1/1 -> Gain/1, [RePr]
  Gain/1 -> Switch5/1
  Divide3/1 -> Product1/1
  [HydD] -> Divide3/2
  Thermal Conductivity/1 -> Divide3/1
  Math Function/1 -> Switch5/2
  [DoL] -> Math Function/1
  Vector Concatenate1/1 -> Calculation1/1
  Prandtl Number/1 -> Vector Concatenate1/2
  Divide/1 -> Vector Concatenate1/1  "ReD"
  Abs Viscosity/1 -> Divide/4
  Divide2/1 -> [DoL]
  TubLen/1 -> Divide2/2
  [HydD] -> Divide2/1
  CrossA/1 -> Divide/3
  HydDia/1 -> Divide/2, [HydD]
  [CoolTemp] -> Thermal Conductivity/1
  FluidTemp/1 -> Abs Viscosity/1, [CoolTemp], Prandtl Number/1
  LPF with IC1/1(y) -> HTC/1  "HTCest"

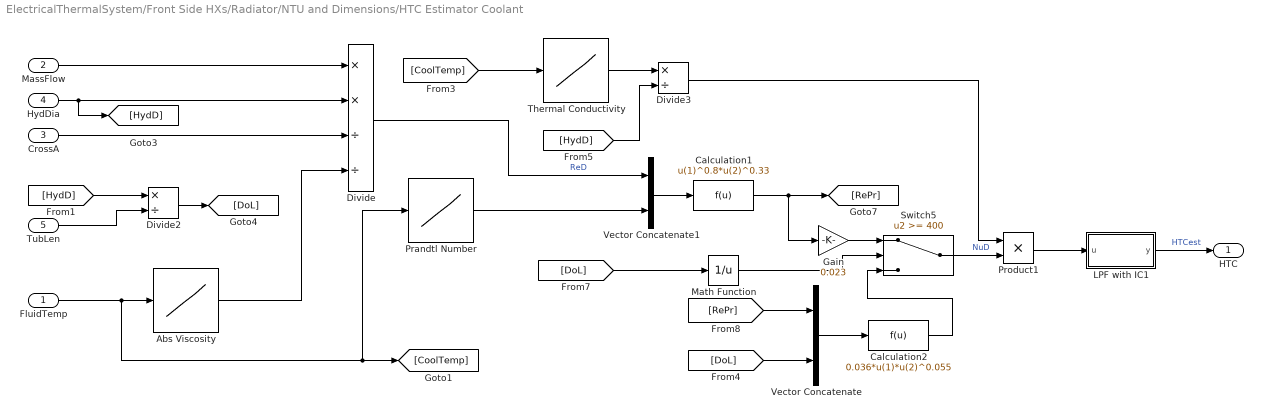
== system ElectricalThermalSystem/Front Side HXs/Radiator/NTU and Dimensions/HTC Estimator Coolant ==
  FluidTemp : Inport
  MassFlow : Inport  Port=2
  CrossA : Inport  Port=3  OutMin=eps
  HydDia : Inport  Port=4
  TubLen : Inport  Port=5
  Abs Viscosity : Lookup_n-D  NumberOfTableDimensions=1  BreakpointsForDimension1=PlntThrCoolCpBpt  Table=PlntThrCoolVisc  ExtrapMethod=Clip  UseLastTableValue=on  InternalRulePriority=Speed  RndMeth=Simplest
  Calculation1 : Fcn  Expr=u(1)^0.8*u(2)^0.33
  Calculation2 : Fcn  Expr=0.036*u(1)*u(2)^0.055
  Divide : Product  Inputs=**//
  Divide2 : Product  Inputs=*/
  Divide3 : Product  Inputs=*/
  Gain : Gain  Gain=0.023
  LPF with IC1 : Subsystem  mask{wc=10, InitCond=10, dataType=off}
      mask prompts: wc "Cutoff frequency, wc [rad/s]"; InitCond "Initial condition, InitCond [same as u]"; dataType "Enforce same input data type"
      mask TypeOptions wc: Cont LPF IC/wc
      mask TypeOptions InitCond: Initial Condition/Value
      mask TypeOptions dataType: Cont LPF IC/dataType
  Math Function : Math  Operator=reciprocal
  Prandtl Number : Lookup_n-D  NumberOfTableDimensions=1  BreakpointsForDimension1=PlntThrCoolCpBpt  Table=PlntThrCoolPrand  ExtrapMethod=Clip  UseLastTableValue=on  InternalRulePriority=Speed  RndMeth=Simplest
  Product1 : Product
  Switch5 : Switch  Threshold=400  SaturateOnIntegerOverflow=off  InputSameDT=off
  Thermal Conductivity : Lookup_n-D  NumberOfTableDimensions=1  BreakpointsForDimension1=PlntThrCoolCpBpt  Table=PlntThrCoolCond  ExtrapMethod=Clip  UseLastTableValue=on  InternalRulePriority=Speed  RndMeth=Simplest
  Vector Concatenate : Concatenate
  Vector Concatenate1 : Concatenate
  HTC : Outport
  wires:
  MassFlow/1 -> Divide/1
  Product1/1 -> LPF with IC1/1(u)
  Switch5/1 -> Product1/2  "NuD"
  Calculation2/1 -> Switch5/3
  Vector Concatenate/1 -> Calculation2/1
  [DoL] -> Vector Concatenate/2
  [RePr] -> Vector Concatenate/1
  Calculation1/1 -> Gain/1, [RePr]
  Gain/1 -> Switch5/1
  Divide3/1 -> Product1/1
  [HydD] -> Divide3/2
  Thermal Conductivity/1 -> Divide3/1
  Math Function/1 -> Switch5/2
  [DoL] -> Math Function/1
  Vector Concatenate1/1 -> Calculation1/1
  Prandtl Number/1 -> Vector Concatenate1/2
  Divide/1 -> Vector Concatenate1/1  "ReD"
  Abs Viscosity/1 -> Divide/4
  Divide2/1 -> [DoL]
  TubLen/1 -> Divide2/2
  [HydD] -> Divide2/1
  CrossA/1 -> Divide/3
  HydDia/1 -> Divide/2, [HydD]
  [CoolTemp] -> Thermal Conductivity/1
  FluidTemp/1 -> Abs Viscosity/1, [CoolTemp], Prandtl Number/1
  LPF with IC1/1(y) -> HTC/1  "HTCest"

== system ElectricalThermalSystem/Heater Battery DCDC Converter/Battery/HTC Estimator Batt/LPF with IC1 ==
  u : Inport
  Cont LPF IC : autolibutils/Cont LPF IC  wc=wc  aMode=1  dataType=off
  Initial Condition : Constant  Value=InitCond  SampleTime=-1
  y : Outport
  wires:
  Cont LPF IC/1 -> y/1
  u/1 -> Cont LPF IC/1
  Initial Condition/1 -> Cont LPF IC/2

== system ElectricalThermalSystem/Heater Battery DCDC Converter/DC-DC Converter/HTC Estimator DCDC/LPF with IC1 ==
  u : Inport
  Cont LPF IC : autolibutils/Cont LPF IC  wc=wc  aMode=1  dataType=off
  Initial Condition : Constant  Value=InitCond  SampleTime=-1
  y : Outport
  wires:
  Cont LPF IC/1 -> y/1
  u/1 -> Cont LPF IC/1
  Initial Condition/1 -> Cont LPF IC/2

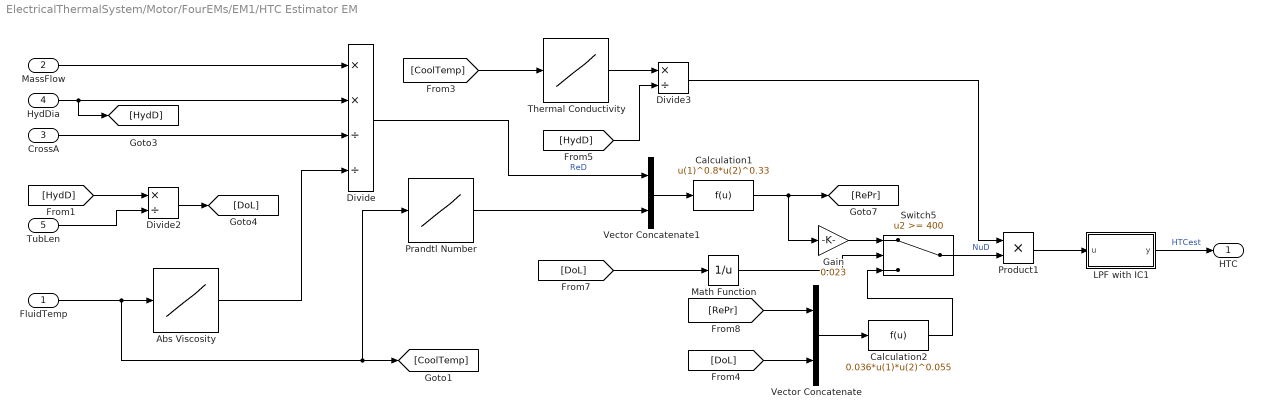
== system ElectricalThermalSystem/Motor/FourEMs/EM1/HTC Estimator EM ==
  FluidTemp : Inport
  MassFlow : Inport  Port=2
  CrossA : Inport  Port=3  OutMin=eps
  HydDia : Inport  Port=4
  TubLen : Inport  Port=5
  Abs Viscosity : Lookup_n-D  NumberOfTableDimensions=1  BreakpointsForDimension1=PlntThrCoolCpBpt  Table=PlntThrCoolVisc  ExtrapMethod=Clip  UseLastTableValue=on  InternalRulePriority=Speed  RndMeth=Simplest
  Calculation1 : Fcn  Expr=u(1)^0.8*u(2)^0.33
  Calculation2 : Fcn  Expr=0.036*u(1)*u(2)^0.055
  Divide : Product  Inputs=**//
  Divide2 : Product  Inputs=*/
  Divide3 : Product  Inputs=*/
  Gain : Gain  Gain=0.023
  LPF with IC1 : Subsystem  mask{wc=10, InitCond=10, dataType=off}
      mask prompts: wc "Cutoff frequency, wc [rad/s]"; InitCond "Initial condition, InitCond [same as u]"; dataType "Enforce same input data type"
      mask TypeOptions wc: Cont LPF IC/wc
      mask TypeOptions InitCond: Initial Condition/Value
      mask TypeOptions dataType: Cont LPF IC/dataType
  Math Function : Math  Operator=reciprocal
  Prandtl Number : Lookup_n-D  NumberOfTableDimensions=1  BreakpointsForDimension1=PlntThrCoolCpBpt  Table=PlntThrCoolPrand  ExtrapMethod=Clip  UseLastTableValue=on  InternalRulePriority=Speed  RndMeth=Simplest
  Product1 : Product
  Switch5 : Switch  Threshold=400  SaturateOnIntegerOverflow=off  InputSameDT=off
  Thermal Conductivity : Lookup_n-D  NumberOfTableDimensions=1  BreakpointsForDimension1=PlntThrCoolCpBpt  Table=PlntThrCoolCond  ExtrapMethod=Clip  UseLastTableValue=on  InternalRulePriority=Speed  RndMeth=Simplest
  Vector Concatenate : Concatenate
  Vector Concatenate1 : Concatenate
  HTC : Outport
  wires:
  LPF with IC1/1(y) -> HTC/1  "HTCest"
  FluidTemp/1 -> Prandtl Number/1, [CoolTemp], Abs Viscosity/1
  [CoolTemp] -> Thermal Conductivity/1
  MassFlow/1 -> Divide/1
  HydDia/1 -> [HydD], Divide/2
  CrossA/1 -> Divide/3
  [HydD] -> Divide2/1
  TubLen/1 -> Divide2/2
  Divide2/1 -> [DoL]
  Abs Viscosity/1 -> Divide/4
  Divide/1 -> Vector Concatenate1/1  "ReD"
  Prandtl Number/1 -> Vector Concatenate1/2
  Vector Concatenate1/1 -> Calculation1/1
  [DoL] -> Math Function/1
  Math Function/1 -> Switch5/2
  Thermal Conductivity/1 -> Divide3/1
  [HydD] -> Divide3/2
  Divide3/1 -> Product1/1
  Gain/1 -> Switch5/1
  Calculation1/1 -> [RePr], Gain/1
  [RePr] -> Vector Concatenate/1
  [DoL] -> Vector Concatenate/2
  Vector Concatenate/1 -> Calculation2/1
  Calculation2/1 -> Switch5/3
  Switch5/1 -> Product1/2  "NuD"
  Product1/1 -> LPF with IC1/1(u)

== system ElectricalThermalSystem/Motor/FourEMs/EM1/Temperature and Heat Flow ==
  HTC : Inport
  CoolTempIn : Inport  Port=2
  EMTemp : Inport  Port=3
  CoolMflw : Inport  Port=4
  JacArea : Inport  Port=5
  Divide2 : Product  Inputs=*/
  Gain4 : Gain  Gain=0.5
  LPF with IC1 : Subsystem  mask{wc=10, InitCond=EnvAirTemp, dataType=off}
      mask prompts: wc "Cutoff frequency, wc [rad/s]"; InitCond "Initial condition, InitCond [same as u]"; dataType "Enforce same input data type"
      mask TypeOptions wc: Cont LPF IC/wc
      mask TypeOptions InitCond: Initial Condition/Value
      mask TypeOptions dataType: Cont LPF IC/dataType
  Minus3 : Sum
  Minus4 : Sum
  Product1 : Product  Inputs=3
  Product2 : Product
  Selector : Selector  InputPortWidth=PlntEMNum  IndexOptions=Index vector (dialog)  Indices=1  OutputSizes=1
  Specific Heat 2 : Lookup_n-D  NumberOfTableDimensions=1  BreakpointsForDimension1=PlntThrCoolCpBpt  Table=PlntThrCoolCp  ExtrapMethod=Clip  UseLastTableValue=on  InternalRulePriority=Speed  RndMeth=Simplest
  Subtract : Sum  Inputs=+-
  div0protect - abs poly4 : autolibutils/div0protect - abs poly  thresh=.001  aMode=1
  BulkCoolTemp : Outport
  Qem : Outport  Port=2
  CoolTempOut : Outport  Port=3
  wires:
  LPF with IC1/1(y) -> BulkCoolTemp/1, [BulkCoolTemp]
  EMTemp/1 -> Selector/1
  HTC/1 -> Product1/1
  Product2/1 -> div0protect - abs poly4/1
  Minus4/1 -> Gain4/1
  Gain4/1 -> LPF with IC1/1(u)
  Minus3/1 -> Minus4/2, CoolTempOut/1
  Product1/1 -> Divide2/1, Qem/1  "Qem"
  JacArea/1 -> Product1/2
  div0protect - abs poly4/1 -> Divide2/2
  Specific Heat 2/1 -> Product2/2
  [BulkCoolTemp] -> Specific Heat 2/1, Subtract/2
  Subtract/1 -> Product1/3
  Selector/1 -> Subtract/1
  Divide2/1 -> Minus3/2
  CoolMflw/1 -> Product2/1
  CoolTempIn/1 -> Minus4/1, Minus3/1
